simulink model "simulink_FCS_SDA"  (R2023a)
settings: Solver=VariableStepAuto  StartTime=0.0  StopTime=3*(1/freqHzSin)  FixedStep=Ts  RelTol=1e-3
InitFcn:
  | % try
  | %     Excel = actxGetRunningServer('Excel.Application');
  | %     Excel.ActiveWorkbook.Save;
  | %     Excel.ActiveWorkbook.Close(false);
  | % catch ExcelFechado
  | % end
StopFcn:
  | % t = table(out.seq, out.t_sim, 'VariableNames', ["Sequência de Vetores","Tempo de Simulação"]);
  | % writetable(t,'C:\Users\jpbru\OneDrive\Documentos\UFSC\COBEP 2023\sequencia_states.xlsx','Sheet','sim_CF_gw')
  | % winopen('C:\Users\jpbru\OneDrive\Documentos\UFSC\COBEP 2023\sequencia_states.xlsx')
  | %
  | % nome_arq = sprintf("gdq_caso-1_7.csv");
  | % writematrix([out.y_d out.y_q out.y_a out.y_b out.y_c out.ref_a out.ref_b out.ref_c],"C:\Users\jpbru\OneDrive\Documentos\MATLAB\CPBM\TrabFinal\Etapa 9 - Setembro2023 -\graficos\"+nome_arq)
  | 
  | sprintf("THD = %.3f", out.thd)
  | sprintf("MSE = %.3f", out.mse)
  | sprintf("Csw = %.0f", out.csw)
  | sprintf("Tempo de Computo = %.3fms", out.tavg*1000)
values from neighbouring files (symbols this model uses):
  Csim = Cf*(1-P/100)    (= 5e-05)    [script_SDA.m]
  freqHzSin = 50    [script_SDA.m]
  Lsim = Lf*(1-P/100)    (= 0.002)    [script_SDA.m]
  N = 2    [script_SDA.m]
  N1 = 1    [script_SDA.m]
  N2 = N-N1+1    (= 2)    [script_SDA.m]
  Niter_max = 32000    [script_SDA.m]
  Rsim = Rl*(1-P/100)    (= 60)    [script_SDA.m]
  Ts = 1/Fs    (= 0.0001)    [script_SDA.m]
  Vdc_sim = Vdc*1    (= 400)    [script_SDA.m]
  Vnoise = 0    [script_SDA.m]
undefined symbols (not defined in the file or in its folder): DiscIntNeverNeededParam, Gamma, H, Lfilter, lSTE, UpsilonT, Vref_pico, W_inv
libraries: dspstat3 x9, spsSeriesRLCBranchLib x9, spsVoltageMeasurementLib x7, spsCurrentMeasurementLib x6, spsIdealSwitchLib x6, spsTHDLib x4, spsabctoAlphaBetaZeroLib x4, simulink x2, spsAlphaBetaZerotoabcLib x1, spsControlledVoltageSourceLib x1, sps_lib x1
settings Model: Creator=jpbru  LastModifiedBy=jpbru
settings SolverCC: AlgebraicLoopSolver=TrustRegion
settings DebuggingCC: UnconnectedInputMsg=warning  UnconnectedOutputMsg=warning  UnconnectedLineMsg=warning
settings ModelReferenceCC: EnableRefExpFcnMdlSchedulingChecks=on

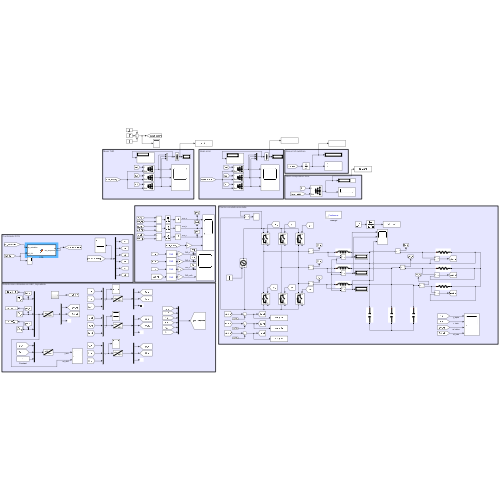
[thumbnail: Simulink's stored preview of the top-level diagram]
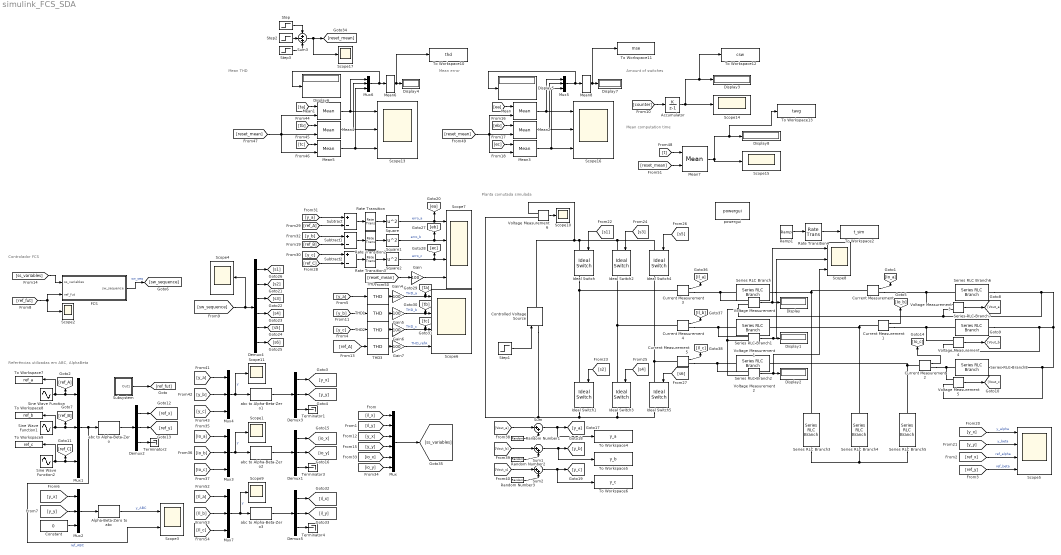
== system simulink_FCS_SDA ==
  note: Planta comutada simulada
  note: Referências utilizadas em ABC, AlphaBeta
  note: Controlador FCS
  note: Mean computation time
  note: Mean error
  note: Amount of switches
  note: Mean THD
  Accumulator : DiscreteIntegrator  IntegratorMethod=Accumulation: Forward Euler  SampleTime=-1  ICPrevOutput=DiscIntNeverNeededParam  ICPrevScaledInput=DiscIntNeverNeededParam
  Alpha-Beta-Zero to abc : spsAlphaBetaZerotoabcLib/Alpha-Beta-Zero to abc
      settings: LibrarySourceBlock=|
      | sps_lib/Control/Alpha-Beta-Zero
      | to abc
  Constant : Constant  Value=0  VectorParams1D=off  SampleTime=-1
  Controlled Voltage Source : spsControlledVoltageSourceLib/Controlled Voltage Source  Initialize=on  Source_Type=DC  Amplitude=Vdc_sim  Phase=0  Frequency=0  Measurements=None
  Current Measurement{,1..5} (6 alike) : spsCurrentMeasurementLib/Current Measurement  PhasorSimulation=off  OutputType=Complex  PSBequivalent=0
  Demux{1..3,5} (4 alike) : Demux  Outputs=3
  Demux4 : Demux  Outputs=6
  Display{,1..8} (9 alike) : Display
      Display8 settings: Format=short_e
  FCS : MATLAB Function  TreatAsAtomicUnit=on  SystemSampleTime=Ts
  Gain{,4..7} (5 alike) : Gain  Gain=100
  Ideal Switch{,1..5} (6 alike) : spsIdealSwitchLib/Ideal Switch  Ron=0.001  Lon=0  IC=0  Rs=1e5  Cs=inf  Measurements=on
  Mean{,1..5,7} (7 alike) : dspstat3/Mean  run=on  reset_popup=Rising edge  directionMode=Each column  dimension=1  roiEnable=off  roiType=Rectangles  roiPortion=Entire ROI  roiOutput=Individual statistics for each ROI  roiFlag=off  roundingMode=Floor  overflowMode=off  outputDataTypeStr=Inherit: Same as accumulator  outputMin=[]  outputMax=[]  outputLastDataTypeStr=Inherit: Same as accumulator
  Mean6 : dspstat3/Mean  run=off  reset_popup=Rising edge  directionMode=Entire input  dimension=1  roiEnable=off  roiType=Rectangles  roiPortion=Entire ROI  roiOutput=Individual statistics for each ROI  roiFlag=off  roundingMode=Floor  overflowMode=off  outputDataTypeStr=Inherit: Same as accumulator  outputMin=[]  outputMax=[]  outputLastDataTypeStr=Inherit: Same as accumulator
  Mean8 : dspstat3/Mean  run=off  reset_popup=Rising edge  directionMode=Entire input  dimension=1  roiEnable=off  roiType=Rectangles  roiPortion=Entire ROI  roiOutput=Individual statistics for each ROI  roiFlag=off  roundingMode=Floor  overflowMode=off  outputDataTypeStr=Inherit: Same as accumulator  outputMin=[]  outputMax=[]  outputLastDataTypeStr=Inherit: Same as accumulator
  Mux : Mux  Inputs=6
  Mux{1..7} (7 alike) : Mux  Inputs=3
  Ramp1 : simulink/Sources/Ramp  slope=1  start=0  InitialOutput=0
  Random Number1 : RandomNumber  Variance=Vnoise  SampleTime=Ts
  Random Number2 : RandomNumber  Variance=Vnoise  SampleTime=Ts
  Random Number3 : RandomNumber  Variance=Vnoise  SampleTime=Ts
  Rate Transition{,2..4} (4 alike) : RateTransition  OutPortSampleTime=Ts
  Scope{1..2,4,9..11,14..15,17} (9 alike) : Scope
  Scope13 : Scope  NumInputPorts=3
  Scope16 : Scope  NumInputPorts=3
  Scope3 : Scope  NumInputPorts=2
  Scope5 : Scope  NumInputPorts=4
  Scope6 : Scope  NumInputPorts=4
  Scope7 : Scope  NumInputPorts=4
  Scope8 : Scope  NumInputPorts=3
  Series RLC Branch : spsSeriesRLCBranchLib/Series RLC Branch  LConnTagsString=__new0  RConnTagsString=__new0  BranchType=L  Resistance=1  Inductance=Lsim  SetiL0=off  InitialCurrent=0  Capacitance=1e-6  Setx0=off  InitialVoltage=0  Measurements=None
  Series RLC Branch1 : spsSeriesRLCBranchLib/Series RLC Branch  LConnTagsString=__new0  RConnTagsString=__new0  BranchType=L  Resistance=1  Inductance=Lsim  SetiL0=off  InitialCurrent=0  Capacitance=1e-6  Setx0=off  InitialVoltage=0  Measurements=None
  Series RLC Branch2 : spsSeriesRLCBranchLib/Series RLC Branch  LConnTagsString=__new0  RConnTagsString=__new0  BranchType=L  Resistance=1  Inductance=Lsim  SetiL0=off  InitialCurrent=0  Capacitance=1e-6  Setx0=off  InitialVoltage=0  Measurements=None
  Series RLC Branch3 : spsSeriesRLCBranchLib/Series RLC Branch  LConnTagsString=__new0  RConnTagsString=__new0  BranchType=C  Resistance=1  Inductance=1e-3  SetiL0=off  InitialCurrent=0  Capacitance=Csim  Setx0=off  InitialVoltage=0  Measurements=None
  Series RLC Branch4 : spsSeriesRLCBranchLib/Series RLC Branch  LConnTagsString=__new0  RConnTagsString=__new0  BranchType=C  Resistance=1  Inductance=1e-3  SetiL0=off  InitialCurrent=0  Capacitance=Csim  Setx0=off  InitialVoltage=0  Measurements=None
  Series RLC Branch5 : spsSeriesRLCBranchLib/Series RLC Branch  LConnTagsString=__new0  RConnTagsString=__new0  BranchType=C  Resistance=1  Inductance=1e-3  SetiL0=off  InitialCurrent=0  Capacitance=Csim  Setx0=off  InitialVoltage=0  Measurements=None
  Series RLC Branch6 : spsSeriesRLCBranchLib/Series RLC Branch  LConnTagsString=__new0  RConnTagsString=__new0  BranchType=R  Resistance=Rsim  Inductance=Lfilter  SetiL0=off  InitialCurrent=0  Capacitance=1e-6  Setx0=off  InitialVoltage=0  Measurements=None
  Series RLC Branch7 : spsSeriesRLCBranchLib/Series RLC Branch  LConnTagsString=__new0  RConnTagsString=__new0  BranchType=R  Resistance=Rsim  Inductance=Lfilter  SetiL0=off  InitialCurrent=0  Capacitance=1e-6  Setx0=off  InitialVoltage=0  Measurements=None
  Series RLC Branch8 : spsSeriesRLCBranchLib/Series RLC Branch  LConnTagsString=__new0  RConnTagsString=__new0  BranchType=R  Resistance=Rsim  Inductance=Lfilter  SetiL0=off  InitialCurrent=0  Capacitance=1e-6  Setx0=off  InitialVoltage=0  Measurements=None
  Sine Wave Function : Sin  Amplitude=Vref_pico  Frequency=2*pi*50  SampleTime=Ts
  Sine Wave Function1 : Sin  Amplitude=Vref_pico  Frequency=2*pi*50  Phase=-2*pi/3  SampleTime=Ts
  Sine Wave Function2 : Sin  Amplitude=Vref_pico  Frequency=2*pi*50  Phase=2*pi/3  SampleTime=Ts
  Square : Math  Operator=square
  Square1 : Math  Operator=square
  Square2 : Math  Operator=square
  Step : Step  Time=(1/freqHzSin)  SampleTime=Ts
  Step1 : Step  Time=0.5  Before=Vdc_sim  After=Vdc_sim  SampleTime=Ts
  Step2 : Step  Time=(1/freqHzSin)+Ts  SampleTime=Ts
  Step3 : Step  Time=(1/freqHzSin)*2  SampleTime=Ts
  Subsystem : Subsystem
  Subtract : Sum  Inputs=+-
  Subtract1 : Sum  Inputs=+-
  Subtract2 : Sum  Inputs=+-
  Sum : Sum  Inputs=|++
  Sum1 : Sum  Inputs=|++
  Sum2 : Sum  Inputs=|++
  Sum3 : Sum  Inputs=+-+
  THD{,1..3} (4 alike) : spsTHDLib/THD  Freq=50  Ts=Ts
  Terminator{1..4} (4 alike) : Terminator
  To Workspace10 : ToWorkspace  VariableName=thd  SampleTime=-1
      settings: MaxDataPoints=1
  To Workspace11 : ToWorkspace  VariableName=mse  SampleTime=-1
      settings: MaxDataPoints=1
  To Workspace12 : ToWorkspace  VariableName=csw  SampleTime=-1
      settings: MaxDataPoints=1
  To Workspace13 : ToWorkspace  VariableName=tavg  SampleTime=-1
      settings: MaxDataPoints=1
  To Workspace2 : ToWorkspace  VariableName=t_sim  SampleTime=Ts
      settings: Save2DSignal=2-D array (concatenate along first dimension)
  To Workspace4 : ToWorkspace  VariableName=y_a  SampleTime=Ts
      settings: Save2DSignal=2-D array (concatenate along first dimension)
  To Workspace5 : ToWorkspace  VariableName=y_b  SampleTime=Ts
      settings: Save2DSignal=2-D array (concatenate along first dimension)
  To Workspace6 : ToWorkspace  VariableName=y_c  SampleTime=Ts
      settings: Save2DSignal=2-D array (concatenate along first dimension)
  To Workspace7 : ToWorkspace  VariableName=ref_a  SampleTime=Ts
      settings: Save2DSignal=2-D array (concatenate along first dimension)
  To Workspace8 : ToWorkspace  VariableName=ref_b  SampleTime=Ts
      settings: Save2DSignal=2-D array (concatenate along first dimension)
  To Workspace9 : ToWorkspace  VariableName=ref_c  SampleTime=Ts
      settings: Save2DSignal=2-D array (concatenate along first dimension)
  Voltage Measurement{,1..6} (7 alike) : spsVoltageMeasurementLib/Voltage Measurement  PhasorSimulation=off  OutputType=Complex  PSBequivalent=0
  abc to Alpha-Beta-Zero{,1..3} (4 alike) : spsabctoAlphaBetaZeroLib/abc to Alpha-Beta-Zero
  powergui : sps_lib/powergui  Priority=1  SimulationMode=Continuous  SampleTime=Ts  frequency=60  Iterations=50  frequencyindice=0  Pbase=100e6  ErrMax=1e-4  UnitsV=kV  UnitsW=MW  buscounter=0  FunctionMessages=off  echomessages=off  EnableUseOfTLC=off  CurrentSourceSwitches=off  DisableSnubberDevices=off  DisableRonSwitches=off  DisableVfSwitches=off  DisplayEquations=off  AutomaticDiscreteSolvers=off  SolverType=Tustin/Backward Euler (TBE)  Interpol=off  ExternalGateDelay=off  methode=off  Ts=100  x0status=blocks  SPID=on  SwTol=0  HookPort=off  NonlinearTolerance=1e-4  nMaxIteration=100  ContinueOnMaxIteration=off  RestoreLinks=warning  ResistiveCurrentMeasurement=off  Frange=[0:2:500]  Ylog=off  Xlog=on  ShowGrid=off  save=off  variable=ZData  structure=0  ZoomFFT=off  StartTime=0.0  cycles=1  DisplayStyle=1  fundamental=60  FreqAxis=off  MaxFrequency=1000  frequencyindicesteady=1  RmsSteady=1  display=off
  wires:
  [ref_y] -> Scope5/4  "ref_beta"
  Sine Wave Function/1 -> Mux1/1, [ref_A], To Workspace7/1
  Sine Wave Function1/1 -> [ref_B], Mux1/2, To Workspace8/1
  Sine Wave Function2/1 -> [ref_C], Mux1/3, To Workspace9/1
  Mux1/1 -> abc to Alpha-Beta-Zero/1, Scope3/2  "ref_ABC"
  [y_x] -> Mux2/1
  [y_y] -> Mux2/2
  Constant/1 -> Mux2/3
  Alpha-Beta-Zero to abc/1 -> Scope3/1  "y_ABC"
  Voltage Measurement2/1 -> Scope8/3, Display2/1
  Voltage Measurement/1 -> Scope8/1, Display/1
  Voltage Measurement3/1 -> [Vout_a]
  Voltage Measurement4/1 -> [Vout_b]
  Voltage Measurement1/1 -> Scope8/2, Display1/1
  Voltage Measurement5/1 -> [Vout_c]
  [y_b] -> Mux4/2
  [y_a] -> Mux4/1
  [y_c] -> Mux4/3
  abc to Alpha-Beta-Zero1/1 -> Demux3/1
  Demux3/1 -> [y_x]
  Demux3/2 -> [y_y]
  [y_x] -> Scope5/1  "y_alpha"
  [y_y] -> Scope5/2  "y_beta"
  Demux3/3 -> Terminator1/1
  [s6] -> Ideal Switch5/1
  [s1] -> Ideal Switch/1
  [s2] -> Ideal Switch1/1
  [s3] -> Ideal Switch2/1
  [s5] -> Ideal Switch4/1
  [s4] -> Ideal Switch3/1
  Demux4/3 -> [s3]
  Demux4/1 -> [s1]
  Demux4/2 -> [s2]
  Demux4/5 -> [s5]
  Demux4/6 -> [s6]
  Demux4/4 -> [s4]
  [sw_sequence] -> Scope4/1, Demux4/1
  FCS/1(sw_sequence) -> [sw_sequence]  "sw_seq"
  [ss_variables] -> FCS/1(ss_variables)
  [ref_x] -> Scope5/3  "ref_alpha"
  Demux2/2 -> [ref_y]
  Demux2/1 -> [ref_x]
  Demux2/3 -> Terminator2/1
  abc to Alpha-Beta-Zero/1 -> Demux2/1
  Mux4/1 -> Scope11/1, abc to Alpha-Beta-Zero1/1  "y"
  Mux2/1 -> Alpha-Beta-Zero to abc/1
  Subsystem/1(Out1) -> [ref_fut]
  [ref_fut] -> FCS/2(ref_fut), Scope2/1
  Voltage Measurement6/1 -> Scope10/1
  [Vout_b] -> Sum1/1
  Sum2/1 -> To Workspace6/1, [y_c]
  Sum/1 -> To Workspace4/1, [y_a]
  Random Number1/1 -> Sum/2
  Random Number2/1 -> Sum1/2
  Random Number3/1 -> Sum2/2
  Sum1/1 -> To Workspace5/1, [y_b]
  [Vout_a] -> Sum/1
  [Vout_c] -> Sum2/1
  [t] -> Mean7/1
  Mean7/1 -> To Workspace13/1, Display8/1, Scope15/1
  [ea] -> Mean/1
  [ec] -> Mean3/1
  Mux5/1 -> Mean8/1, Display5/1
  Mean/1 -> Mux5/1, Scope16/1
  Mean3/1 -> Mux5/3, Scope16/3
  Mean2/1 -> Mux5/2, Scope16/2
  [eb] -> Mean2/1
  THD/1 -> Gain4/1
  Square1/1 -> [eb], Scope7/2  "erro_b"
  [y_b] -> THD1/1
  [ref_B] -> Subtract1/2
  Gain5/1 -> [tb], Scope6/2  "THD_b"
  [y_c] -> Subtract2/1
  [y_b] -> Subtract1/1
  [ref_C] -> Subtract2/2
  [y_a] -> Subtract/1
  [ref_A] -> THD3/1
  THD1/1 -> Gain5/1
  Gain7/1 -> Scope6/4  "THD_refA"
  Subtract1/1 -> Rate Transition2/1
  THD2/1 -> Gain6/1
  Square2/1 -> [ec], Scope7/3  "erro_c"
  [ref_A] -> Subtract/2
  THD3/1 -> Gain7/1
  Gain6/1 -> [tc], Scope6/3  "THD_c"
  Subtract2/1 -> Rate Transition3/1
  [y_a] -> THD/1
  Subtract/1 -> Rate Transition/1
  Square/1 -> [ea], Scope7/1  "erro_a"
  [y_c] -> THD2/1
  Gain4/1 -> [ta], Scope6/1  "THD_a"
  Accumulator/1 -> To Workspace12/1, Display3/1, Scope14/1
  [counter] -> Accumulator/1
  [tc] -> Mean5/1
  [ta] -> Mean1/1
  Mean5/1 -> Mux6/3, Scope13/3
  Mean4/1 -> Mux6/2, Scope13/2
  [tb] -> Mean4/1
  Mux6/1 -> Display6/1, Mean6/1
  Mean1/1 -> Mux6/1, Scope13/1
  Rate Transition/1 -> Square/1
  Rate Transition2/1 -> Square1/1
  Rate Transition3/1 -> Square2/1
  [reset_mean] -> Mean1/2, Mean5/2, Mean4/2
  [reset_mean] -> Mean3/2, Mean2/2, Mean/2
  [reset_mean] -> Gain/1
  Gain/1 -> Scope7/4
  [reset_mean] -> Mean7/2
  Mean6/1 -> To Workspace10/1, Display4/1
  Mean8/1 -> To Workspace11/1, Display7/1
  Step1/1 -> Controlled Voltage Source/1
  Ramp1/1 -> Rate Transition4/1
  Rate Transition4/1 -> To Workspace2/1
  Step/1 -> Sum3/1
  Step3/1 -> Sum3/3
  Step2/1 -> Sum3/2
  Sum3/1 -> Scope17/1, [reset_mean]
  [il_x] -> Mux/1
  [il_y] -> Mux/2
  [io_y] -> Mux/6
  [io_x] -> Mux/5
  [y_y] -> Mux/4
  [y_x] -> Mux/3
  Current Measurement/1 -> [Io_a]
  Current Measurement1/1 -> [Io_b]
  Current Measurement2/1 -> [Io_c]
  Demux1/3 -> Terminator3/1
  abc to Alpha-Beta-Zero2/1 -> Demux1/1
  Mux3/1 -> Scope1/1, abc to Alpha-Beta-Zero2/1  "y"
  Demux1/1 -> [io_x]
  [Io_c] -> Mux3/3
  [Io_a] -> Mux3/1
  Demux1/2 -> [io_y]
  [Io_b] -> Mux3/2
  Mux7/1 -> Scope9/1, abc to Alpha-Beta-Zero3/1  "y"
  abc to Alpha-Beta-Zero3/1 -> Demux5/1
  [Il_c] -> Mux7/3
  [Il_b] -> Mux7/2
  Demux5/1 -> [il_x]
  Demux5/2 -> [il_y]
  [Il_a] -> Mux7/1
  Demux5/3 -> Terminator4/1
  Mux/1 -> [ss_variables]
  Current Measurement5/1 -> [Il_c]
  Current Measurement4/1 -> [Il_b]
  Current Measurement3/1 -> [Il_a]
  connections:
  Ideal Switch3/LConn1 -- Current Measurement4/LConn1 -- Ideal Switch2/RConn1
  Series RLC Branch/LConn1 -- Current Measurement3/RConn1 -- Voltage Measurement/LConn1
  Series RLC Branch6/RConn1 -- Voltage Measurement2/LConn2 -- Voltage Measurement1/LConn2 -- Voltage Measurement/LConn2 -- Voltage Measurement3/LConn2 -- Voltage Measurement4/LConn2 -- Series RLC Branch7/RConn1 -- Voltage Measurement5/LConn2 -- Series RLC Branch8/RConn1
  Series RLC Branch2/LConn1 -- Current Measurement5/RConn1 -- Voltage Measurement2/LConn1
  Series RLC Branch3/RConn1 -- Series RLC Branch5/RConn1 -- Series RLC Branch4/RConn1
  Voltage Measurement3/LConn1 -- Current Measurement/RConn1 -- Series RLC Branch6/LConn1
  Series RLC Branch5/LConn1 -- Current Measurement2/LConn1 -- Series RLC Branch2/RConn1
  Series RLC Branch4/LConn1 -- Current Measurement1/LConn1 -- Series RLC Branch1/RConn1
  Ideal Switch/LConn1 -- Controlled Voltage Source/RConn1 -- Voltage Measurement6/LConn1 -- Ideal Switch4/LConn1 -- Ideal Switch2/LConn1
  Ideal Switch1/RConn1 -- Controlled Voltage Source/LConn1 -- Voltage Measurement6/LConn2 -- Ideal Switch5/RConn1 -- Ideal Switch3/RConn1
  Series RLC Branch/RConn1 -- Series RLC Branch3/LConn1 -- Current Measurement/LConn1
  Series RLC Branch7/LConn1 -- Current Measurement1/RConn1 -- Voltage Measurement4/LConn1
  Series RLC Branch8/LConn1 -- Current Measurement2/RConn1 -- Voltage Measurement5/LConn1
  Ideal Switch/RConn1 -- Current Measurement3/LConn1 -- Ideal Switch1/LConn1
  Series RLC Branch1/LConn1 -- Current Measurement4/RConn1 -- Voltage Measurement1/LConn1
  Ideal Switch5/LConn1 -- Current Measurement5/LConn1 -- Ideal Switch4/RConn1

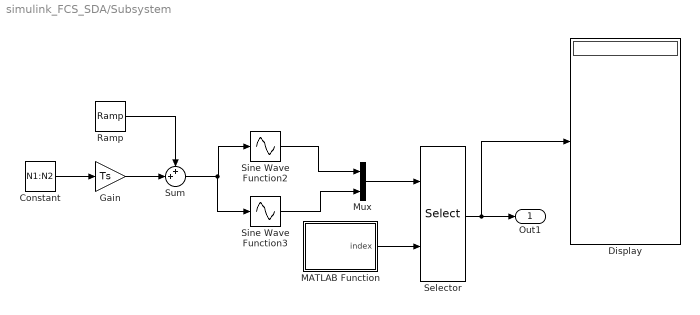
== system simulink_FCS_SDA/Subsystem ==
  Constant : Constant  Value=N1:N2
  Display : Display
  Gain : Gain  Gain=Ts
  MATLAB Function : MATLAB Function  TreatAsAtomicUnit=on
  Mux : Mux  Inputs=2
  Ramp : simulink/Sources/Ramp  slope=1  start=0  InitialOutput=0
  Selector : Selector  InputPortWidth=2*N  IndexOptions=Index vector (port)  Indices=[1:N]  OutputSizes=1
  Sine Wave Function2 : Sin  TimeSource=Use external signal  Amplitude=Vref_pico  Frequency=2*pi*50  SampleTime=Ts
  Sine Wave Function3 : Sin  TimeSource=Use external signal  Amplitude=Vref_pico  Frequency=2*pi*50  Phase=-pi/2  SampleTime=Ts
  Sum : Sum  Inputs=++|
  Out1 : Outport
  wires:
  Sine Wave Function2/1 -> Mux/1
  Sum/1 -> Sine Wave Function3/1, Sine Wave Function2/1
  Ramp/1 -> Sum/1
  Gain/1 -> Sum/2
  Constant/1 -> Gain/1
  Sine Wave Function3/1 -> Mux/2
  Mux/1 -> Selector/1
  MATLAB Function/1(index) -> Selector/2
  Selector/1 -> Display/1, Out1/1

== matlab function simulink_FCS_SDA/FCS ==
  settings: updateMethod=DISCRETE  sampleTime=Ts
  data: ss_variables input; sw_sequence output; ref_fut input; UpsilonT parameter; Gamma parameter; lSTE parameter; W_inv parameter; H parameter; Niter_max parameter
%function[variáveis que envia pra fora do bloco na simulação] = fcn(entradas(com conexões físicas) e parâmetros(que são pegos da workspace))
function sw_sequence  = fcn(ss_variables, ref_fut, UpsilonT, Gamma, lSTE, W_inv, H, Niter_max) 
persistent t total_iter uabc_k_1 x_k %variáveis que mantém o valor entre os loops
if isempty(t) %caso t ainda não tenha valor definido
    t = 0; %o primeiro loop assume t=0
    total_iter = 0; %variável que vai contar quantos loops são feitos para o cálculo de control
    uabc_k_1 = [0 0 0]';
else %caso não seja o primeiro loop
    t = t + 1; %t vai incrementando em cada loop
end
x_k = ss_variables;
Yref = ref_fut;

%% Unconstrained solution calculation
F_k=UpsilonT*(Gamma*x_k-Yref)-lSTE*uabc_k_1;
U_unc=-W_inv*F_k;
%U_unc = 4*(rand(p,1)-0.5); % To generate randomly
%U_unc = min(u_max+1, max(u_min-1, U_unc)); % Limit unconstrained values
U_bar_unc = H*U_unc;          % Center of the sphere in the transformed space

%% Initial Vector U_ini -> Only for SDA
% U_ini = zeros(p,1);               % Null vector
U_ini=round(U_unc);    % Babai
for k =1 : p
   if (U_ini(k,1)<u_min)
       U_ini(k,1)=u_min;
   end
   if (U_ini(k,1)>u_max)
       U_ini(k,1)=u_max;
   end
end

Niter=0; %variable that shows the number of iterations
d=zeros((p+1),1); 
U_k=zeros(p,1); 
U_op=U_ini; 

%% Initial Radius of Sphere (Squared value)
Rs2 = ceil((norm(U_bar_unc - H*U_ini))^2); %rounds the squared value to the nearest integer towards infinity
Rs2_ini = Rs2;


%% Sphere Decoding  Algorithm %%%%%%%%%%%%%%%%%%%%%%%%%%%%
%%%%%%%%%%%%%%%%%%%%%%%%%%%%%%%%%%%%%%%%%%%%%%%%%%%%%%%%%%%%%%%%%%%%%%%%%%
%tic
i = 0; C=0;
% i is the index of input vector dimension (i = 1 -> phase A; i = 2 -> B; i = 3 -> C)
% C is the index of input vector value (C = 0 or 1, i.e., the switching states)

while (i >=0) &&(Niter < Niter_max) % Optimal or early termination
    i=i+1; %i goes to the first layer
    j = u_min + C; %as u_min is 0 and C is 0(at the beggining), j starts in 0 - That is the value that will be considered in the i-th layer
    
    if j <= u_max %if j <= 1
        U_k(i) = j; %The vector U_k in the layer i is j (1st: i = 1, j = 0, U_k(1) = 0)
        d(i+1) = ((H(i,1:i)*U_k(1:i) - U_bar_unc(i))^2 + d(i)); %compute the accumulated distance (among the layers) between the computed U_k and the unconstrained solution, both in the transformed space, and stores in i+1                                 
        Niter=Niter+1; %increase in 1 the number of iterations
        if d(i+1) > Rs2 % If the distance is greater than the radius of the sphere
            i=i-1; C=C+1; %i decreases by 1 and C increases by 1 (this way, the U(i) = 1 will be tested, once that, in the next iteration, i=i+1)
        else            % If the distance is lower than the radius of the sphere
            if i==p           % If all the entire sequence has been computed
               U_op = U_k;    % Update the optimal solution
               Rs2 = d(i+1);  % Save the current squared radius    
               i=i-1; C=C+1; %i decreases by 1 and C increases by 1 in order to test U(i) = 1
            else        % Keep exploring sequence
               C=0;         %resets C
            end % if i==p         
        end % if d(i+1) > Rs2      
    else  %if j > 1
        i=i-2; % i decreases by 2 (if j>1 it means that U(i)=0 and U(i)=1 was computed, so it has to go back to the previous layer. Note that -2 is here because i=i+1 is in the next iteration)
        if i>=0 %if i >= 0, there are options to compute
            C=U_k(i+1) - u_min + 1; 
        end %if i>=0
    end % j <= u_max  
end % While
%toc
uabc_k_1 = U_op(1:3,1);
total_iter = total_iter+Niter;
%%%%%%%%%%%%%%%%%%%%%%%% End of Sphere Decoding  Algorithm %%%%%%%%%%%%%%%
%%%%%%%%%%%%%%%%%%%%%%%%%%%%%%%%%%%%%%%%%%%%%%%%%%%%%%%%%%%%%%%%%%%%%%%%%%

%% Apply the computed switching states
sw_sequence = zeros(6,1); %vetor que define o estado de cada uma das 6 chaves para aplicar nessa amostra
for aux = 1:3 %loop para definir o vetor
    sw_sequence(2*aux-1) = uabc_k_1(aux); 
    sw_sequence(2*aux) = not(uabc_k_1(aux));
end

end

== matlab function simulink_FCS_SDA/Subsystem/MATLAB Function ==
  data: index output; N parameter
function index = fcn(N)
ind = zeros(2*N,1);
counter = 0;
for i=1:2:2*N
    counter = counter + 1;
    ind(i)=counter;
    ind(i+1)=counter+N;
end

index = ind;
